simulink library "SLNS"  (R2023a)
settings: Solver=VariableStepAuto  StartTime=0.0  StopTime=10.0  RelTol=1e-3
libraries: $bdroot x11
settings Model: Creator=Szalay  LastModifiedBy=Szalay
settings DebuggingCC: UnconnectedInputMsg=warning  UnconnectedOutputMsg=warning  UnconnectedLineMsg=warning
settings ModelReferenceCC: EnableRefExpFcnMdlSchedulingChecks=on
settings RTWCC: DLArmComputeVersion=19.05

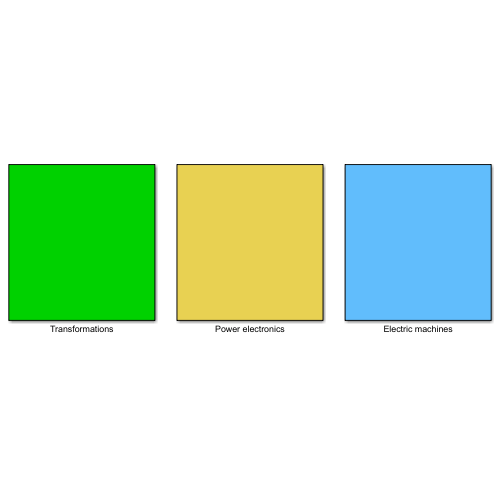
[thumbnail: Simulink's stored preview of the top-level diagram]
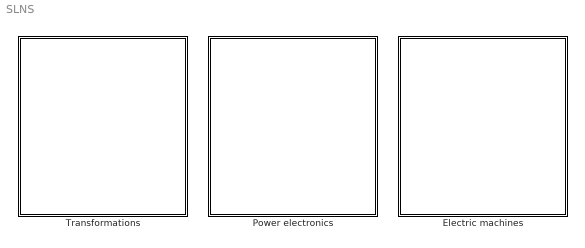
== system SLNS ==
  Electric machines : Subsystem
  Power electronics : Subsystem
  Transformations : Subsystem

== system SLNS/Electric machines ==
  NL-PMSM : Subsystem  mask(Permanent magnet synchronous motor){varZp=2, varRs=0.45, varF_PM=24.83, varLd=142.8, varLq=188.4, varG_0=0.125, varB=6.329e-3, varJ=200, i_d0=0, i_q0=0}
      mask prompts: varZp "Number of pole-pairs"; varRs "Phase resistance [Ω]"; varF_PM "Permanent magnet flux-linkage [mWb]"; varLd "D-direction self-inductance [μH]"; varLq "Q-direction self-inductance [μH]"; varG_0 "Polarity dependent saliency coefficient [μH/A]"; varB "Friction coefficient [N m s/rad]"; varJ "Inertia [g cm²]"; i_d0 "Initial d-direction current [A]"; i_q0 "Initial q-direction current [A]"
      mask help: <p>The d-q model of a <b>permanent magnet synchronous motor</b>, extended with a quadratic flux linkage-phase current equation.</p>
      mask init:
      | L_dd = varLd * 1e-6;
      | L_qq = varLq * 1e-6;
      | 
      | G_ddd = -9/4 * varG_0 * 1e-6;
      | G_dqq = -3/4 * varG_0 * 1e-6;
      | G_qdq = -3/4 * varG_0 * 1e-6;
      | 
      | F_PM = varF_PM * 1e-3;
      | 
      | R = varRs;
      | J = varJ * 1e-3 * 1e-4;	% gcm^2 -> kgm^2
      | B = varB;
      | 
      | z_P = varZp;
      mask DialogControl Container5 Prompt: Machine parameters
      mask DialogControl ElectricalParameters Prompt: Electrical parameters
      mask DialogControl MechanicalParameters Prompt: Mechanical parameters
      mask DialogControl Container6 Prompt: Initial values
      mask Display:
      | port_label('input', 1, '\itu_a', 'texmode', 'on');
      | port_label('input', 2, '\itu_b', 'texmode', 'on');
      | port_label('input', 3, '\itu_c', 'texmode', 'on');
      | port_label('input', 4, '\itM_L', 'texmode', 'on');
      | port_label('input', 5, '{\it\vartheta_M}(0)', 'texmode', 'on');
      | 
      | port_label('output', 1, '\iti_a', 'texmode', 'on');
      | port_label('output', 2, '\iti_b', 'texmode', 'on');
      | port_label('output', 3, '\iti_c', 'texmode', 'on');
      | port_label('output', 4, '\it\omega_M', 'texmode', 'on');
      | port_label('output', 5, '\it\vartheta_M', 'texmode', 'on');
      | 
      | % Felirat
      | text(0.5, 0.5, '{\bfNL-PMSM}', ...
      | 	'HorizontalAlignment', 'center', ...
      | 	'Interpreter', 'tex' ...
      | 	);

== system SLNS/Power electronics ==
  Bipolar triangle wave : Subsystem  mask(Bipolar triangle wave){f=10000, q=0}
      mask prompts: f "Frequency [Hz]"; q "Phase [rad]"
      mask help: Bipolar triangle wave of specified frecency and phase. The amplitude is 1.
      mask DialogControl ParameterGroupVar Prompt: Settings
      mask Display: port_label('output', 1, '{\itc}', 'texmode', 'on');
  Three-phase PWM : Subsystem  mask(Three-phase PWM){f=40000}
      mask prompts: f "Frequency [Hz]"
      mask help: <b>Three-phase pulse width modulation</b> with variable DC-link potentials and natural modulation.
      mask DialogControl ParameterGroupVar Prompt: Settings
      mask Display:
      | port_label('input', 1, '{\itU_{TP}}', 'texmode', 'on');
      | 
      | port_label('input', 2, '{\itu_a}', 'texmode', 'on');
      | port_label('input', 3, '{\itu_b}', 'texmode', 'on');
      | port_label('input', 4, '{\itu_c}', 'texmode', 'on');
      | 
      | port_label('input', 5, '{\itU_{TN}}', 'texmode', 'on');
      | 
      | port_label('output', 1, '{\itu_{a0}}', 'texmode', 'on');
      | port_label('output', 2, '{\itu_{b0}}', 'texmode', 'on');
      | port_label('output', 3, '{\itu_{c0}}', 'texmode', 'on');

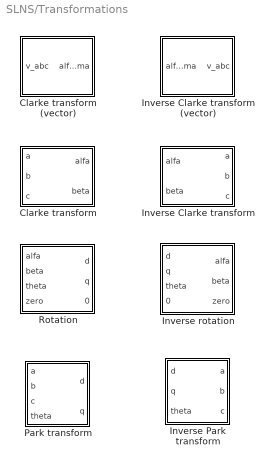
== system SLNS/Transformations ==
  Clarke transform : Subsystem  mask(Clarke-átalakítás){ShowZeroSequence=off}
      mask prompts: ShowZeroSequence "A zérusrendű összetevő használata"
      mask help: <p>Koordináta átalakítás az állórészhez rögzített <i>abc</i> háromfázisú koordinátarendszerből az <i>αβ</i>0 kétfázisúba.
      mask init:
      | SL.ToggleOutport('zero', ShowZeroSequence);
      mask DialogControl ParameterGroupVar Prompt: Beállítások
      mask Display:
      | % Bemenetek
      | port_label('input', 1, '{\ita}', 'texmode', 'on');
      | port_label('input', 2, '{\itb}', 'texmode', 'on');
      | port_label('input', 3, '{\itc}', 'texmode', 'on');
      | 
      | % Kimenetek
      | port_label('output', 1, '{\it\alpha}', 'texmode', 'on');
      | port_label('output', 2, '{\it\beta}', 'texmode', 'on');
      | 
      | if SL.IsOutport('zero')
      | 	port_label('output', 3, '{\it\gamma}', 'texmode', 'on');
      | end
      | 
      | % Felirat
      | text(0.5, 0.5, '{\bfC}', ...
      | 	'HorizontalAlignment', 'center', ...
      | 	'Interpreter', 'tex' ...
      | 	);
  Clarke transform (vector) : Subsystem  mask(Clarke-átalakítás){}
      mask help: <p>Koordináta átalakítás az állórészhez rögzített <i>abc</i> háromfázisú koordinátarendszerből az <i>αβγ</i> kétfázisúba.
      mask Display:
      | % Bemenetek
      | port_label('input', 1, '{\itv̱_{abc}}', 'texmode', 'on');
      | 
      | % Kimenetek
      | port_label('output', 1, '{\itv̱_{\alpha\beta\gamma}}', 'texmode', 'on');
      | 
      | % Felirat
      | % A mátrixjelölést próbáltam aláhúzással is {C̲̲}
      | text(0.5, 0.5, '{\bf C}', ...
      | 	'HorizontalAlignment', 'center', ...
      | 	'Interpreter', 'tex' ...
      | 	);
  Inverse Clarke transform : Subsystem  mask(Inverz Clarke-átalakítás){ShowZeroSequence=off}
      mask prompts: ShowZeroSequence "A zérusrendű összetevő használata"
      mask help: <p>Koordináta átalakítás az állórészhez rögzített <i>αβγ</i> kétfázisú koordinátarendszerből az <i>abc</i> háromfázisúba.
      mask init:
      | SL.ToggleInport('zero', ShowZeroSequence);
      mask DialogControl ParameterGroupVar Prompt: Beállítások
      mask Display:
      | port_label('input', 1, '{\it\alpha}', 'texmode', 'on');
      | port_label('input', 2, '{\it\beta}', 'texmode', 'on');
      | 
      | if( strcmp(get_param([gcb '/zero'], 'BlockType'), 'Inport') )
      | 	port_label('input', 3, '{\it\gamma}', 'texmode', 'on');
      | end
      | 
      | port_label('output', 1, '\ita', 'texmode', 'on');
      | port_label('output', 2, '\itb', 'texmode', 'on');
      | port_label('output', 3, '\itc', 'texmode', 'on');
      | 
      | % Felirat
      | text(0.5, 0.5, '{\bfC}^{-1}', ...
      | 	'HorizontalAlignment', 'center', ...
      | 	'Interpreter', 'tex' ...
      | 	);
  Inverse Clarke transform (vector) : Subsystem  mask(Clarke-átalakítás){}
      mask help: <p>Koordináta átalakítás az állórészhez rögzített <i>abc</i> háromfázisú koordinátarendszerből az <i>αβγ</i> kétfázisúba.
      mask Display:
      | % Bemenetek
      | port_label('input', 1, '{\itv̱_{\alpha\beta\gamma}}', 'texmode', 'on');
      | 
      | % Kimenetek
      | port_label('output', 1, '{\itv̱_{abc}}', 'texmode', 'on');
      | 
      | % Felirat
      | text(0.5, 0.5, '{\bfC^{-1}}', ...
      | 	'HorizontalAlignment', 'center', ...
      | 	'Interpreter', 'tex' ...
      | 	);
  Inverse Park transform : Subsystem  mask(Inverse Park transform){cbZero=off}
      mask prompts: cbZero "Show zero sequence component"
      mask help: Conversion from the the rotating dq/dq0 reference frame to the stationary abc refrence frame.
      mask init:
      | switch cbZero
      | 	case 'on'
      | 		if strcmp(get_param([gcb, '/0'], 'BlockType'), 'Constant')
      | 			SL.BlockSwap([gcb, '/0'], 'built-in/Inport');
      | 		end
      | 	case 'off'
      | 		if strcmp(get_param([gcb, '/0'], 'BlockType'), 'Inport')
      | 			SL.BlockSwap([gcb, '/0'], 'built-in/Constant');
      | 			set_param([gcb, '/0'], 'Value', num2str(0));
      | 		end
      | 	otherwise
      | 		disp(cbZero);
      | end
      mask DialogControl ParameterGroupVar Prompt: Settings
      mask Display:
      | port_label('input', 1, '\itd', 'texmode', 'on');
      | port_label('input', 2, '\itq', 'texmode', 'on');
      | port_label('input', 3, '\it\vartheta', 'texmode', 'on');
      | 
      | if( strcmp(get_param([gcb, '/0'], 'BlockType'), 'Inport') )
      | 	port_label('input', 4, '0', 'texmode', 'on');
      | end
      | 
      | port_label('output', 1, '\ita', 'texmode', 'on');
      | port_label('output', 2, '\itb', 'texmode', 'on');
      | port_label('output', 3, '\itc', 'texmode', 'on');
      | 
      | % Felirat
      | % A "-1"-es kitevő előtt egy vékony szóköz van.
      | text(0.5, 0.5, '{\bfT}^{ -1}(\vartheta)', ...
      | 	'HorizontalAlignment', 'center', ...
      | 	'Interpreter', 'tex' ...
      | 	);
  Inverse rotation : Subsystem  mask{cbZero=on}
      mask prompts: cbZero "Zérusrendű összetevők mutatása"
      mask init:
      | % Inicializáció
      | 
      | switch cbZero
      | 	case 'on'
      | 		if strcmp(get_param([gcb, '/zero'], 'BlockType'), 'Terminator')
      | 			SL.BlockSwap([gcb, '/zero'], 'built-in/Outport');
      | 		end
      | 		if strcmp(get_param([gcb, '/0'], 'BlockType'), 'Constant')
      | 			SL.BlockSwap([gcb, '/0'], 'built-in/Inport');
      | 		end
      | 	case 'off'
      | 		if strcmp(get_param([gcb '/zero'], 'BlockType'), 'Outport')
      | 			SL.BlockSwap([gcb, '/zero'], 'built-in/Terminator');
      | 		end
      | 		if strcmp(get_param([gcb, '/0'], 'BlockType'), 'Inport')
      | 			SL.BlockSwap([gcb, '/0'], 'built-in/Constant');
      | 			set_param([gcb, '/0'], 'Value', num2str(0));
      | 		end
      | 	otherwise
      | 		disp(cbZero);
      | end
      mask Display:
      | port_label('input', 1, '\itd', 'texmode', 'on');
      | port_label('input', 2, '\itq', 'texmode', 'on');
      | port_label('input', 3, '\it\vartheta', 'texmode', 'on');
      | 
      | if( strcmp(get_param([gcb '/0'], 'BlockType'), 'Inport') )
      | 	port_label('input', 4, '0', 'texmode', 'on');
      | end
      | 
      | port_label('output', 1, '\it\alpha', 'texmode', 'on');
      | port_label('output', 2, '\it\beta', 'texmode', 'on');
      | 
      | if( strcmp(get_param([gcb '/zero'], 'BlockType'), 'Outport') )
      | 	port_label('output', 3, '\it\gamma', 'texmode', 'on');
      | end
      | 
      | % Felirat
      | text(0.5, 0.5, '{\bfR}^{-1}(-\vartheta)', ...
      | 	'HorizontalAlignment', 'center', ...
      | 	'Interpreter', 'tex' ...
      | 	);
  Park transform : Subsystem  mask(Park transform){cbZero=off}
      mask prompts: cbZero "Show zero sequence component"
      mask help: Conversion from the stationary abc refrence frame to the rotating dq/dq0 reference frame.
      mask init:
      | switch cbZero
      | 	case 'on'
      | 		if strcmp(get_param([gcb, '/0'], 'BlockType'), 'Terminator')
      | 			SL.BlockSwap([gcb, '/0'], 'built-in/Outport');
      | 		end
      | 	case 'off'
      | 		if strcmp(get_param([gcb '/0'], 'BlockType'), 'Outport')
      | 			SL.BlockSwap([gcb, '/0'], 'built-in/Terminator');
      | 		end
      | 	otherwise
      | 		disp(cbZero);
      | end
      mask DialogControl ParameterGroupVar Prompt: Settings
      mask Display:
      | port_label('input', 1, '{\ita}', 'texmode', 'on');
      | port_label('input', 2, '{\itb}', 'texmode', 'on');
      | port_label('input', 3, '{\itc}', 'texmode', 'on');
      | port_label('input', 4, '{\it\vartheta}', 'texmode', 'on');
      | 
      | port_label('output', 1, '{\itd}', 'texmode', 'on');
      | port_label('output', 2, '{\itq}', 'texmode', 'on');
      | 
      | if( strcmp(get_param([gcb '/0'], 'BlockType'), 'Outport') )
      | 	port_label('output', 3, '0', 'texmode', 'on');
      | end
      | 
      | % Felirat
      | text(0.5, 0.5, '{\bfT}(\vartheta)', ...
      | 	'HorizontalAlignment', 'center', ...
      | 	'Interpreter', 'tex' ...
      | 	);
  Rotation : Subsystem  mask{cbShowZeroSequence=on}
      mask prompts: cbShowZeroSequence "Zérusrendű összetevők mutatása"
      mask init:
      | % Inicializáció
      | 
      | switch cbShowZeroSequence
      | 	case 'on'
      | 		if strcmp(get_param([gcb, '/0'], 'BlockType'), 'Terminator')
      | 			SL.BlockSwap([gcb, '/0'], 'built-in/Outport');
      | 		end
      | 		if strcmp(get_param([gcb, '/zero'], 'BlockType'), 'Constant')
      | 			SL.BlockSwap([gcb, '/zero'], 'built-in/Inport');
      | 		end
      | 	case 'off'
      | 		if strcmp(get_param([gcb '/0'], 'BlockType'), 'Outport')
      | 			SL.BlockSwap([gcb, '/0'], 'built-in/Terminator');
      | 		end
      | 		if strcmp(get_param([gcb, '/zero'], 'BlockType'), 'Inport')
      | 			SL.BlockSwap([gcb, '/zero'], 'built-in/Constant');
      | 			set_param([gcb, '/zero'], 'Value', num2str(0));
      | 		end
      | 	otherwise
      | 		disp(cbShowZeroSequence);
      | end
      mask Display:
      | port_label('input', 1, '\it\alpha', 'texmode', 'on');
      | port_label('input', 2, '\it\beta', 'texmode', 'on');
      | port_label('input', 3, '\it\vartheta', 'texmode', 'on');
      | 
      | if( strcmp(get_param([gcb '/zero'], 'BlockType'), 'Inport') )
      | 	port_label('input', 4, '\it\gamma', 'texmode', 'on');
      | end
      | 
      | port_label('output', 1, '\itd', 'texmode', 'on');
      | port_label('output', 2, '\itq', 'texmode', 'on');
      | 
      | if( strcmp(get_param([gcb '/0'], 'BlockType'), 'Outport') )
      | 	port_label('output', 3, '0', 'texmode', 'on');
      | end
      | 
      | % Felirat
      | text(0.5, 0.5, '{\bfR}(-{\it\vartheta})', ...
      | 	'HorizontalAlignment', 'center', ...
      | 	'Interpreter', 'tex' ...
      | 	);

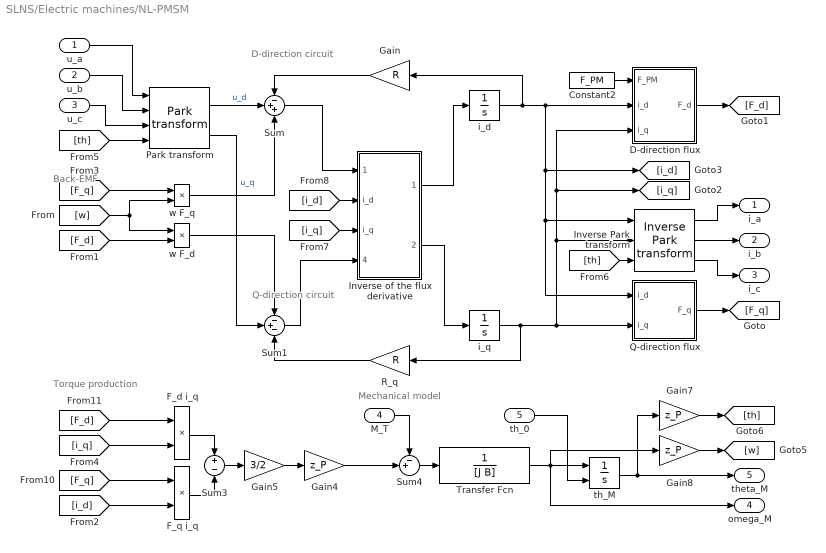
== system SLNS/Electric machines/NL-PMSM ==
  note: Torque production
  note: Back-EMF
  note: Q-direction circuit
  note: D-direction circuit
  note: Mechanical model
  u_a : Inport
  u_b : Inport  Port=2
  u_c : Inport  Port=3
  M_T : Inport  Port=4
  th_0 : Inport  Port=5
  Constant2 : Constant  Value=F_PM
  D-direction flux : Subsystem
      mask Display:
      | % Bemenetek
      | port_label('input', 1, '\Psi^{\itPM}', 'texmode', 'on');
      | port_label('input', 2, '\iti_d', 'texmode', 'on');
      | port_label('input', 3, '\iti_q', 'texmode', 'on');
      | 
      | % Kimenetek
      | port_label('output', 1, '\Psi_{\itd}', 'texmode', 'on');
  F_d i_q : Product
  F_q i_q : Product
  Gain : Gain  Gain=R
  Gain4 : Gain  Gain=z_P
  Gain5 : Gain  Gain=3/2
  Gain7 : Gain  Gain=z_P
  Gain8 : Gain  Gain=z_P
  Inverse Park transform : $bdroot/Transformations/Inverse Park transform  cbZero=off
  Inverse of the flux derivative : Subsystem
      mask Display:
      | % Bemenetek
      | port_label('input', 1, 'd\Psi_{\itd} /d{\itt}', 'texmode', 'on');
      | port_label('input', 2, '\iti_d', 'texmode', 'on');
      | port_label('input', 3, '\iti_q', 'texmode', 'on');
      | port_label('input', 4, 'd\Psi_{\itq} /d{\itt}', 'texmode', 'on');
      | 
      | % Kimenetek
      | port_label('output', 1, 'd{\iti_d} /d{\itt}', 'texmode', 'on');
      | port_label('output', 2, 'd{\iti_q} /d{\itt}', 'texmode', 'on');
  Park transform : $bdroot/Transformations/Park transform  cbZero=off
  Q-direction flux : Subsystem
      mask Display:
      | % Bemenetek
      | port_label('input', 1, '\iti_d', 'texmode', 'on');
      | port_label('input', 2, '\iti_q', 'texmode', 'on');
      | 
      | % Kimenetek
      | port_label('output', 1, '\Psi_{\itq}', 'texmode', 'on');
  R_q : Gain  Gain=R
  Sum : Sum  Inputs=-++
  Sum1 : Sum  Inputs=-+-
  Sum3 : Sum  Inputs=+|-
  Sum4 : Sum  Inputs=-+|
  Transfer Fcn : TransferFcn  Denominator=[J B]
  i_d : Integrator  InitialCondition=i_d0
  i_q : Integrator  InitialCondition=i_q0
  th_M : Integrator  InitialConditionSource=external
  w F_d : Product
  w F_q : Product
  i_a : Outport  VectorParamsAs1DForOutWhenUnconnected=off
  i_b : Outport  Port=2  VectorParamsAs1DForOutWhenUnconnected=off
  i_c : Outport  Port=3  VectorParamsAs1DForOutWhenUnconnected=off
  omega_M : Outport  Port=4  VectorParamsAs1DForOutWhenUnconnected=off
  theta_M : Outport  Port=5  VectorParamsAs1DForOutWhenUnconnected=off
  wires:
  Sum4/1 -> Transfer Fcn/1
  [i_q] -> Inverse of the flux derivative/3(i_q)
  [i_d] -> Inverse of the flux derivative/2(i_d)
  Inverse of the flux derivative/1(di_d/dt) -> i_d/1
  Inverse of the flux derivative/2(di_q/dt) -> i_q/1
  th_M/1 -> Gain7/1, theta_M/1
  Inverse Park transform/3 -> i_c/1
  Inverse Park transform/2 -> i_b/1
  Inverse Park transform/1 -> i_a/1
  [th] -> Inverse Park transform/3
  Transfer Fcn/1 -> Gain8/1, th_M/1, omega_M/1
  Gain8/1 -> [w]
  Gain7/1 -> [th]
  [th] -> Park transform/4
  th_0/1 -> th_M/2
  M_T/1 -> Sum4/1
  Gain4/1 -> Sum4/2
  Gain5/1 -> Gain4/1
  Sum3/1 -> Gain5/1
  F_q i_q/1 -> Sum3/2
  F_d i_q/1 -> Sum3/1
  [i_d] -> F_q i_q/2
  [i_q] -> F_d i_q/2
  [F_q] -> w F_q/1
  [w] -> w F_q/2, w F_d/1
  [F_d] -> w F_d/2
  w F_q/1 -> Sum/3
  Park transform/2 -> Sum1/2  "u_q"
  Q-direction flux/1(F_q) -> [F_q]
  i_d/1 -> D-direction flux/2(i_d), Inverse Park transform/1, Q-direction flux/1(i_d), [i_d], Gain/1
  Gain/1 -> Sum/1
  Park transform/1 -> Sum/2  "u_d"
  u_c/1 -> Park transform/3
  u_b/1 -> Park transform/2
  u_a/1 -> Park transform/1
  Constant2/1 -> D-direction flux/1(F_PM)
  D-direction flux/1(F_d) -> [F_d]
  i_q/1 -> Inverse Park transform/2, [i_q], D-direction flux/3(i_q), Q-direction flux/2(i_q), R_q/1
  Sum/1 -> Inverse of the flux derivative/1(dF_d/dt)
  Sum1/1 -> Inverse of the flux derivative/4(dF_q/dt)
  [F_q] -> F_q i_q/1
  R_q/1 -> Sum1/3
  w F_d/1 -> Sum1/1
  [F_d] -> F_d i_q/1

== system SLNS/Power electronics/Bipolar triangle wave ==
  Cosine : Sin  Frequency=2*pi*f  Phase=q+pi/2  SampleTime=0
  Fcn : Fcn  Expr=asin(u)/(pi/2)
  Out1 : Outport  VectorParamsAs1DForOutWhenUnconnected=off
  wires:
  Fcn/1 -> Out1/1
  Cosine/1 -> Fcn/1

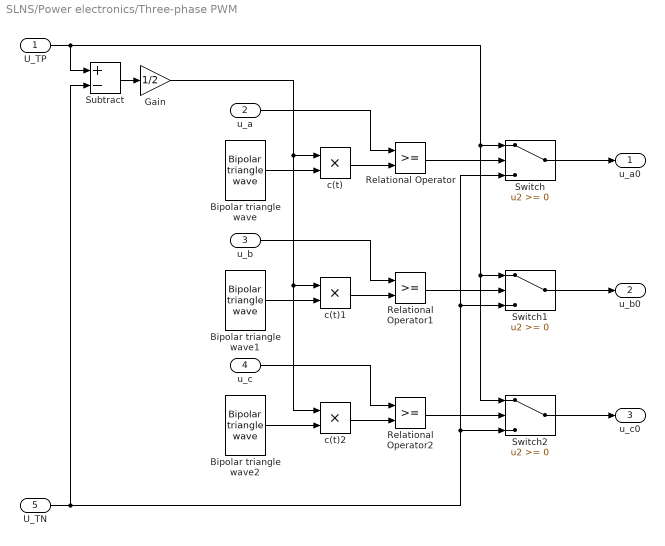
== system SLNS/Power electronics/Three-phase PWM ==
  U_TP : Inport
  u_a : Inport  Port=2
  u_b : Inport  Port=3
  u_c : Inport  Port=4
  U_TN : Inport  Port=5
  Bipolar triangle wave : $bdroot/Power electronics/Bipolar triangle wave  f=f  q=pi
  Bipolar triangle wave1 : $bdroot/Power electronics/Bipolar triangle wave  f=f  q=pi
  Bipolar triangle wave2 : $bdroot/Power electronics/Bipolar triangle wave  f=f  q=pi
  Gain : Gain  Gain=1/2
  Relational Operator : RelationalOperator  OutDataTypeStr=boolean  InputSameDT=off
  Relational Operator1 : RelationalOperator  OutDataTypeStr=boolean  InputSameDT=off
  Relational Operator2 : RelationalOperator  OutDataTypeStr=boolean  InputSameDT=off
  Subtract : Sum  Inputs=+-
  Switch : Switch  SaturateOnIntegerOverflow=off  InputSameDT=off
  Switch1 : Switch  SaturateOnIntegerOverflow=off  InputSameDT=off
  Switch2 : Switch  SaturateOnIntegerOverflow=off  InputSameDT=off
  c(t) : Product  RndMeth=Zero
  c(t)1 : Product  RndMeth=Zero
  c(t)2 : Product  RndMeth=Zero
  u_a0 : Outport  VectorParamsAs1DForOutWhenUnconnected=off
  u_b0 : Outport  Port=2  VectorParamsAs1DForOutWhenUnconnected=off
  u_c0 : Outport  Port=3  VectorParamsAs1DForOutWhenUnconnected=off
  wires:
  Gain/1 -> c(t)/1, c(t)1/1, c(t)2/1
  Subtract/1 -> Gain/1
  U_TN/1 -> Subtract/2, Switch1/3, Switch/3, Switch2/3
  Switch2/1 -> u_c0/1
  u_c/1 -> Relational Operator2/1
  Relational Operator2/1 -> Switch2/2
  c(t)2/1 -> Relational Operator2/2
  Bipolar triangle wave2/1 -> c(t)2/2
  Switch1/1 -> u_b0/1
  u_b/1 -> Relational Operator1/1
  Relational Operator1/1 -> Switch1/2
  c(t)1/1 -> Relational Operator1/2
  Bipolar triangle wave1/1 -> c(t)1/2
  Switch/1 -> u_a0/1
  u_a/1 -> Relational Operator/1
  Relational Operator/1 -> Switch/2
  c(t)/1 -> Relational Operator/2
  U_TP/1 -> Switch2/1, Switch1/1, Switch/1, Subtract/1
  Bipolar triangle wave/1 -> c(t)/2

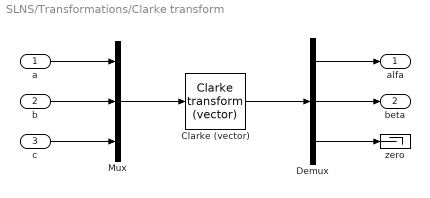
== system SLNS/Transformations/Clarke transform ==
  a : Inport
  b : Inport  Port=2
  c : Inport  Port=3
  Clarke (vector) : $bdroot/Transformations/Clarke transform (vector)
  Demux : Demux  Outputs=3
  Mux : Mux  Inputs=3
  zero : Terminator
  alfa : Outport  VectorParamsAs1DForOutWhenUnconnected=off
  beta : Outport  Port=2
  wires:
  c/1 -> Mux/3
  b/1 -> Mux/2
  a/1 -> Mux/1
  Mux/1 -> Clarke (vector)/1
  Clarke (vector)/1 -> Demux/1
  Demux/2 -> beta/1
  Demux/1 -> alfa/1
  Demux/3 -> zero/1

== system SLNS/Transformations/Clarke transform (vector) ==
  v_abc : Inport
  Fcn0 : Fcn  Expr=1/3*(u(1) + u(2) + u(3))
  FcnA : Fcn  Expr=2/3*(1*u(1) - 0.5*u(2) - 0.5*u(3))
  FcnB : Fcn  Expr=2/3*(sqrt(3)/2*u(2) - sqrt(3)/2*u(3))
  Mux1 : Mux  Inputs=3
  alfa-beta-gamma : Outport  VectorParamsAs1DForOutWhenUnconnected=off
  wires:
  Mux1/1 -> alfa-beta-gamma/1
  Fcn0/1 -> Mux1/3
  FcnA/1 -> Mux1/1
  v_abc/1 -> FcnA/1, FcnB/1, Fcn0/1
  FcnB/1 -> Mux1/2

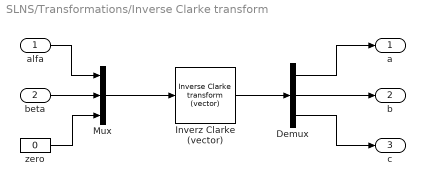
== system SLNS/Transformations/Inverse Clarke transform ==
  alfa : Inport
  beta : Inport  Port=2
  Demux : Demux  Outputs=3
  Inverz Clarke (vector) : $bdroot/Transformations/Inverse Clarke transform (vector)
  Mux : Mux  Inputs=3
  zero : Constant  Value=0
  a : Outport  VectorParamsAs1DForOutWhenUnconnected=off
  b : Outport  Port=2  VectorParamsAs1DForOutWhenUnconnected=off
  c : Outport  Port=3  VectorParamsAs1DForOutWhenUnconnected=off
  wires:
  alfa/1 -> Mux/1
  beta/1 -> Mux/2
  zero/1 -> Mux/3
  Mux/1 -> Inverz Clarke (vector)/1
  Inverz Clarke (vector)/1 -> Demux/1
  Demux/2 -> b/1
  Demux/1 -> a/1
  Demux/3 -> c/1

== system SLNS/Transformations/Inverse Clarke transform (vector) ==
  alfa-beta-gamma : Inport
  FcnA : Fcn  Expr=(1*u(1) + 0*u(2) + 1*u(3))
  FcnB : Fcn  Expr=(-0.5*u(1) + sqrt(3)/2*u(2) + 1*u(3))
  FcnC : Fcn  Expr=(-0.5*u(1) - sqrt(3)/2*u(2) + 1*u(3))
  Mux : Mux  Inputs=3
  v_abc : Outport  VectorParamsAs1DForOutWhenUnconnected=off
  wires:
  alfa-beta-gamma/1 -> FcnB/1, FcnC/1, FcnA/1
  FcnA/1 -> Mux/1
  FcnB/1 -> Mux/2
  FcnC/1 -> Mux/3
  Mux/1 -> v_abc/1

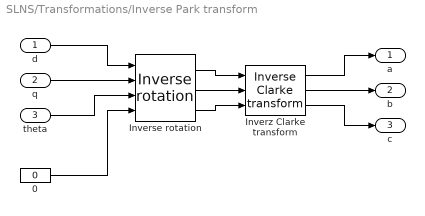
== system SLNS/Transformations/Inverse Park transform ==
  d : Inport
  q : Inport  Port=2
  theta : Inport  Port=3
  0 : Constant  Value=0
  Inverse rotation : $bdroot/Transformations/Inverse rotation  cbZero=on
  Inverz Clarke transform : $bdroot/Transformations/Inverse Clarke transform  ShowZeroSequence=on
  a : Outport  VectorParamsAs1DForOutWhenUnconnected=off
  b : Outport  Port=2  VectorParamsAs1DForOutWhenUnconnected=off
  c : Outport  Port=3  VectorParamsAs1DForOutWhenUnconnected=off
  wires:
  0/1 -> Inverse rotation/4
  Inverz Clarke transform/1 -> a/1
  Inverz Clarke transform/2 -> b/1
  Inverz Clarke transform/3 -> c/1
  d/1 -> Inverse rotation/1
  Inverse rotation/1 -> Inverz Clarke transform/1
  Inverse rotation/2 -> Inverz Clarke transform/2
  q/1 -> Inverse rotation/2
  theta/1 -> Inverse rotation/3
  Inverse rotation/3 -> Inverz Clarke transform/3

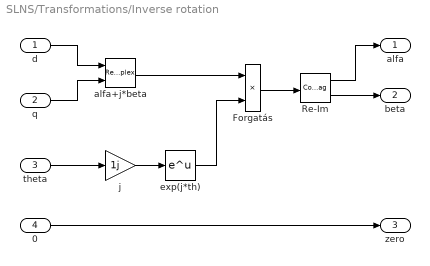
== system SLNS/Transformations/Inverse rotation ==
  d : Inport
  q : Inport  Port=2
  theta : Inport  Port=3
  0 : Inport  Port=4
  Forgatás : Product  RndMeth=Zero
  Re-Im : ComplexToRealImag
  alfa+j*beta : RealImagToComplex
  exp(j*th) : Math  SignedPower=on
  j : Gain  Gain=1j
  alfa : Outport  VectorParamsAs1DForOutWhenUnconnected=off
  beta : Outport  Port=2  VectorParamsAs1DForOutWhenUnconnected=off
  zero : Outport  Port=3  VectorParamsAs1DForOutWhenUnconnected=off
  wires:
  exp(j*th)/1 -> Forgatás/2
  alfa+j*beta/1 -> Forgatás/1
  Forgatás/1 -> Re-Im/1
  theta/1 -> j/1
  Re-Im/1 -> alfa/1
  d/1 -> alfa+j*beta/1
  q/1 -> alfa+j*beta/2
  j/1 -> exp(j*th)/1
  Re-Im/2 -> beta/1
  0/1 -> zero/1

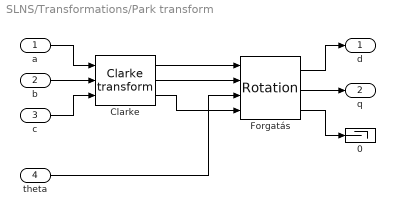
== system SLNS/Transformations/Park transform ==
  a : Inport
  b : Inport  Port=2
  c : Inport  Port=3
  theta : Inport  Port=4
  0 : Terminator
  Clarke : $bdroot/Transformations/Clarke transform  ShowZeroSequence=on
  Forgatás : $bdroot/Transformations/Rotation  cbShowZeroSequence=on
  d : Outport  VectorParamsAs1DForOutWhenUnconnected=off
  q : Outport  Port=2  VectorParamsAs1DForOutWhenUnconnected=off
  wires:
  Forgatás/3 -> 0/1
  Forgatás/2 -> q/1
  Forgatás/1 -> d/1
  b/1 -> Clarke/2
  a/1 -> Clarke/1
  c/1 -> Clarke/3
  Clarke/1 -> Forgatás/1
  Clarke/2 -> Forgatás/2
  Clarke/3 -> Forgatás/4
  theta/1 -> Forgatás/3

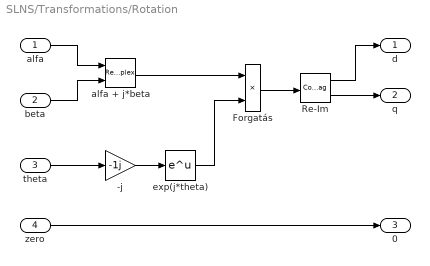
== system SLNS/Transformations/Rotation ==
  alfa : Inport
  beta : Inport  Port=2
  theta : Inport  Port=3
  zero : Inport  Port=4
  -j : Gain  Gain=-1j
  Forgatás : Product  RndMeth=Zero
  Re-Im : ComplexToRealImag
  alfa + j*beta : RealImagToComplex
  exp(j*theta) : Math  SignedPower=on
  d : Outport  VectorParamsAs1DForOutWhenUnconnected=off
  q : Outport  Port=2  VectorParamsAs1DForOutWhenUnconnected=off
  0 : Outport  Port=3
  wires:
  exp(j*theta)/1 -> Forgatás/2
  Re-Im/2 -> q/1
  Forgatás/1 -> Re-Im/1
  -j/1 -> exp(j*theta)/1
  theta/1 -> -j/1
  alfa + j*beta/1 -> Forgatás/1
  beta/1 -> alfa + j*beta/2
  Re-Im/1 -> d/1
  alfa/1 -> alfa + j*beta/1
  zero/1 -> 0/1

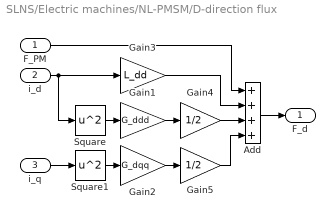
== system SLNS/Electric machines/NL-PMSM/D-direction flux ==
  F_PM : Inport
  i_d : Inport  Port=2
  i_q : Inport  Port=3
  Add : Sum  Inputs=++++
  Gain1 : Gain  Gain=G_ddd
  Gain2 : Gain  Gain=G_dqq
  Gain3 : Gain  Gain=L_dd
  Gain4 : Gain  Gain=1/2
  Gain5 : Gain  Gain=1/2
  Square : Math  Operator=square
  Square1 : Math  Operator=square
  F_d : Outport
  wires:
  Gain3/1 -> Add/2
  F_PM/1 -> Add/1
  Add/1 -> F_d/1
  i_q/1 -> Square1/1
  i_d/1 -> Gain3/1, Square/1
  Square1/1 -> Gain2/1
  Square/1 -> Gain1/1
  Gain2/1 -> Gain5/1
  Gain1/1 -> Gain4/1
  Gain4/1 -> Add/3
  Gain5/1 -> Add/4

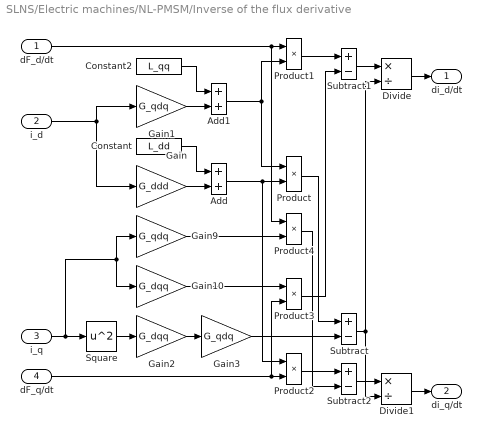
== system SLNS/Electric machines/NL-PMSM/Inverse of the flux derivative ==
  dF_d/dt : Inport
  i_d : Inport  Port=2
  i_q : Inport  Port=3
  dF_q/dt : Inport  Port=4
  Add : Sum
  Add1 : Sum
  Constant : Constant  Value=L_dd
  Constant2 : Constant  Value=L_qq
  Divide : Product  Inputs=*/
  Divide1 : Product  Inputs=*/
  Gain : Gain  Gain=G_ddd
  Gain1 : Gain  Gain=G_qdq
  Gain10 : Gain  Gain=G_dqq
  Gain2 : Gain  Gain=G_dqq
  Gain3 : Gain  Gain=G_qdq
  Gain9 : Gain  Gain=G_qdq
  Product{,1..4} (5 alike) : Product
  Square : Math  Operator=square
  Subtract : Sum  Inputs=+-
  Subtract1 : Sum  Inputs=+-
  Subtract2 : Sum  Inputs=+-
  di_d/dt : Outport
  di_q/dt : Outport  Port=2
  wires:
  Divide1/1 -> di_q/dt/1
  Divide/1 -> di_d/dt/1
  Gain9/1 -> Product4/2
  i_q/1 -> Square/1, Gain9/1, Gain10/1
  dF_q/dt/1 -> Product2/2, Product3/2
  Subtract2/1 -> Divide1/1
  Subtract1/1 -> Divide/1
  Subtract/1 -> Divide1/2, Divide/2
  Gain10/1 -> Product3/1
  dF_d/dt/1 -> Product1/1, Product4/1
  Product3/1 -> Subtract1/2
  Add1/1 -> Product/1, Product1/2
  Product1/1 -> Subtract1/1
  Product4/1 -> Subtract2/2
  Add/1 -> Product/2, Product2/1
  Product2/1 -> Subtract2/1
  i_d/1 -> Gain/1, Gain1/1
  Gain/1 -> Add/2
  Constant/1 -> Add/1
  Constant2/1 -> Add1/1
  Gain1/1 -> Add1/2
  Square/1 -> Gain2/1
  Gain2/1 -> Gain3/1
  Product/1 -> Subtract/1
  Gain3/1 -> Subtract/2

== system SLNS/Electric machines/NL-PMSM/Q-direction flux ==
  i_d : Inport
  i_q : Inport  Port=2
  Add : Sum
  Gain1 : Gain  Gain=G_qdq
  Gain3 : Gain  Gain=L_qq
  Product : Product
  F_q : Outport
  wires:
  Gain1/1 -> Add/1
  i_d/1 -> Product/1
  i_q/1 -> Product/2, Gain3/1
  Add/1 -> F_q/1
  Gain3/1 -> Add/2
  Product/1 -> Gain1/1
